simulink model "Mission_Supervisor"  (R2019b)
settings: Solver=FixedStepAuto  StartTime=0.0  StopTime=inf  FixedStep=0.025  RelTol=1e-3  EnableMultiTasking=on
InitFcn:
  | global clientID;
  | clientID=-1;
libraries: dspindex x4
settings Model: EnablePacing=on  Creator=Kleber Cabral  LastModifiedBy=Kleber Cabral
settings DataIOCC: SaveFormat=Array  ReturnWorkspaceOutputs=off
settings OptimizationCC: LifeSpan=inf
settings DebuggingCC: SolverPrmCheckMsg=warning  SFUnexpectedBacktrackingDiag=warning  SFNoUnconditionalDefaultTransitionDiag=warning  ArithmeticOperatorsInVariantConditions=warning
settings HardwareCC: ProdBitPerPointer=32  ProdBitPerSizeT=32  ProdBitPerPtrDiffT=32  ProdLargestAtomicFloat=None  ProdIntDivRoundTo=Undefined  ProdEndianess=Unspecified  ProdWordSize=32  ProdHWDeviceType=32-bit Generic
settings ModelReferenceCC: PropagateSignalLabelsOutOfModel=off
settings SFSimCC: SimUseLocalCustomCode=off  CustomCodeUndefinedFunction=UseInterfaceOnly
settings RTWCC: RTWUseLocalCustomCode=off
settings CodeAppCC: StateflowObjectComments=on
settings GRTTargetCC: TargetLangStandard=C89/C90 (ANSI)  GeneratePreprocessorConditionals=Disable all
settings ConfigComp: CovMetricSettings=dw  CovHtmlReporting=on  CovSaveCumulativeToWorkspaceVar=on  CovSaveSingleToWorkspaceVar=on  CovExternalEMLEnable=off  CovSFcnEnable=off

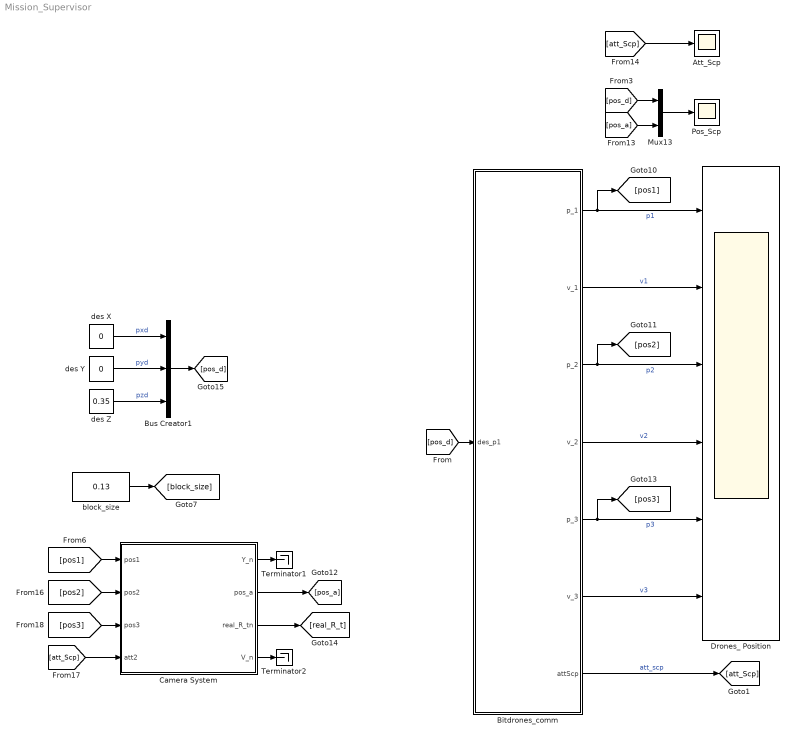
== system Mission_Supervisor ==
  Att_Scp : Scope
  Bitdrones_comm : Subsystem
  Bus Creator1 : BusCreator  Inputs=3
  Camera System : Subsystem
  Drones_ Position : Scope  NumInputPorts=6
  Mux13 : Mux  Inputs=2
  Pos_Scp : Scope
  Terminator1 : Terminator
  Terminator2 : Terminator
  block_size : Constant  Value=0.13
  des X : Constant  Value=0
  des Y : Constant  Value=0
  des Z : Constant  Value=0.35
  wires:
  des X/1 -> Bus Creator1/1  "pxd"
  des Y/1 -> Bus Creator1/2  "pyd"
  des Z/1 -> Bus Creator1/3  "pzd"
  block_size/1 -> [block_size]
  Bitdrones_comm/4(v_2) -> Drones_ Position/4  "v2"
  Bitdrones_comm/2(v_1) -> Drones_ Position/2  "v1"
  Bitdrones_comm/1(p_1) -> [pos1], Drones_ Position/1  "p1"
  Bitdrones_comm/3(p_2) -> [pos2], Drones_ Position/3  "p2"
  Bitdrones_comm/7(attScp) -> [att_Scp]  "att_scp"
  Bitdrones_comm/5(p_3) -> [pos3], Drones_ Position/5  "p3"
  Bitdrones_comm/6(v_3) -> Drones_ Position/6  "v3"
  [att_Scp] -> Att_Scp/1
  [pos_d] -> Mux13/1
  Mux13/1 -> Pos_Scp/1
  [pos_a] -> Mux13/2
  [att_Scp] -> Camera System/4(att2)
  [pos2] -> Camera System/2(pos2)
  Camera System/3(real_R_tn) -> [real_R_t]
  [pos1] -> Camera System/1(pos1)
  [pos3] -> Camera System/3(pos3)
  Camera System/2(pos_a) -> [pos_a]
  Camera System/4(V_n) -> Terminator2/1
  Camera System/1(Y_n) -> Terminator1/1
  Bus Creator1/1 -> [pos_d]
  [pos_d] -> Bitdrones_comm/1(des_p1)

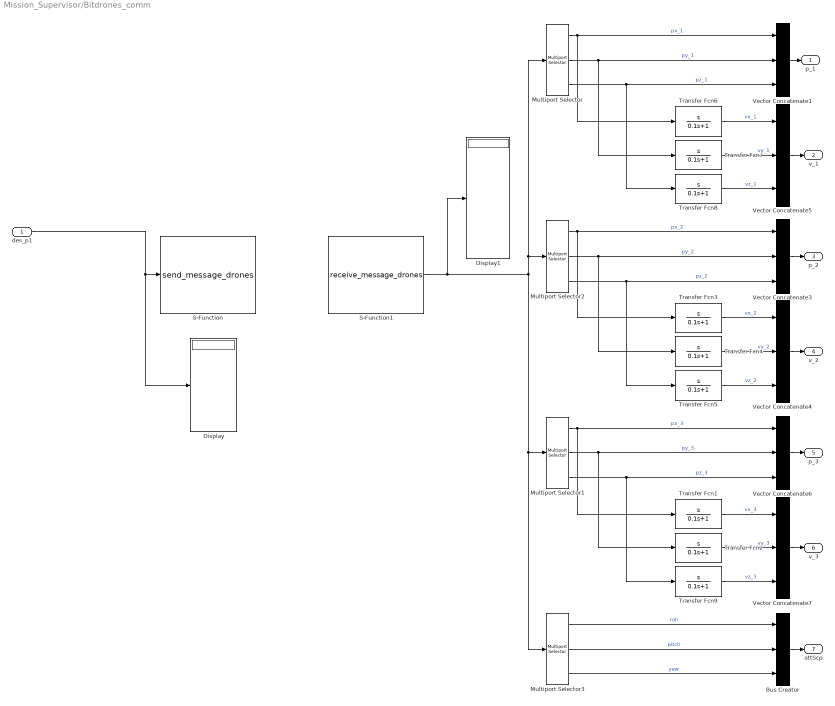
== system Mission_Supervisor/Bitdrones_comm ==
  des_p1 : Inport
  Bus Creator : BusCreator  Inputs=3
  Display : Display
      settings: Decimation=3
  Display1 : Display
      settings: Decimation=3
  Multiport Selector : dspindex/Multiport Selector  rowsOrCols=Rows  idxCellArray={1,2,3}  idxErrMode=Clip Index
  Multiport Selector1 : dspindex/Multiport Selector  rowsOrCols=Rows  idxCellArray={7,8,9}  idxErrMode=Clip Index
  Multiport Selector2 : dspindex/Multiport Selector  rowsOrCols=Rows  idxCellArray={4,5,6}  idxErrMode=Clip Index
  Multiport Selector3 : dspindex/Multiport Selector  rowsOrCols=Rows  idxCellArray={10,11,12}  idxErrMode=Clip Index
  S-Function : S-Function  FunctionName=send_message_drones  SFunctionDeploymentMode=off  EnableBusSupport=off
  S-Function1 : S-Function  FunctionName=receive_message_drones  SFunctionDeploymentMode=off  EnableBusSupport=off
  Transfer Fcn{1..9} (9 alike) : TransferFcn  Numerator=[1 0]  Denominator=[0.1 1]
  Vector Concatenate{1,3..7} (6 alike) : Concatenate  NumInputs=3
  p_1 : Outport
  v_1 : Outport  Port=2
  p_2 : Outport  Port=3
  v_2 : Outport  Port=4
  p_3 : Outport  Port=5
  v_3 : Outport  Port=6
  attScp : Outport  Port=7
  wires:
  Multiport Selector/1 -> Vector Concatenate1/1, Transfer Fcn6/1  "px_1"
  Multiport Selector/2 -> Vector Concatenate1/2, Transfer Fcn7/1  "py_1"
  Multiport Selector/3 -> Vector Concatenate1/3, Transfer Fcn8/1  "pz_1"
  Multiport Selector2/1 -> Vector Concatenate3/1, Transfer Fcn3/1  "px_2"
  Multiport Selector2/2 -> Vector Concatenate3/2, Transfer Fcn4/1  "py_2"
  Multiport Selector2/3 -> Transfer Fcn5/1, Vector Concatenate3/3  "pz_2"
  des_p1/1 -> Display/1, S-Function/1
  Transfer Fcn4/1 -> Vector Concatenate4/2  "vy_2"
  Transfer Fcn5/1 -> Vector Concatenate4/3  "vz_2"
  Vector Concatenate1/1 -> p_1/1
  Vector Concatenate3/1 -> p_2/1
  Vector Concatenate4/1 -> v_2/1
  Transfer Fcn3/1 -> Vector Concatenate4/1  "vx_2"
  Transfer Fcn6/1 -> Vector Concatenate5/1  "vx_1"
  Vector Concatenate5/1 -> v_1/1
  Transfer Fcn8/1 -> Vector Concatenate5/3  "vz_1"
  Transfer Fcn7/1 -> Vector Concatenate5/2  "vy_1"
  Transfer Fcn1/1 -> Vector Concatenate7/1  "vx_3"
  Vector Concatenate7/1 -> v_3/1
  Vector Concatenate6/1 -> p_3/1
  Transfer Fcn9/1 -> Vector Concatenate7/3  "vz_3"
  Transfer Fcn2/1 -> Vector Concatenate7/2  "vy_3"
  Multiport Selector1/3 -> Vector Concatenate6/3, Transfer Fcn9/1  "pz_3"
  Multiport Selector1/2 -> Transfer Fcn2/1, Vector Concatenate6/2  "py_3"
  Multiport Selector1/1 -> Transfer Fcn1/1, Vector Concatenate6/1  "px_3"
  Multiport Selector3/2 -> Bus Creator/2  "pitch"
  Multiport Selector3/3 -> Bus Creator/3  "yaw"
  Bus Creator/1 -> attScp/1
  S-Function1/1 -> Display1/1, Multiport Selector/1, Multiport Selector2/1, Multiport Selector3/1, Multiport Selector1/1
  Multiport Selector3/1 -> Bus Creator/1  "roll"

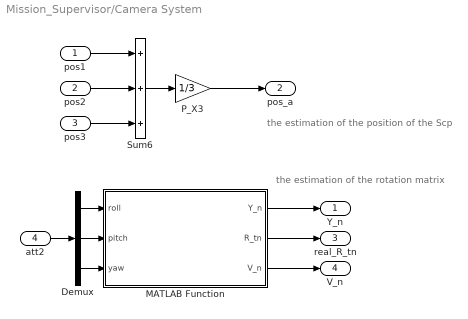
== system Mission_Supervisor/Camera System ==
  note: the estimation of the rotation matrix
  note: the estimation of the position of the Scp
  pos1 : Inport
  pos2 : Inport  Port=2
  pos3 : Inport  Port=3
  att2 : Inport  Port=4
  Demux : Demux  Outputs=3
  MATLAB Function : MATLAB Function  TreatAsAtomicUnit=on
  P_X3 : Gain  Gain=1/3
  Sum6 : Sum  Inputs=+++
  Y_n : Outport  VectorParamsAs1DForOutWhenUnconnected=off
  pos_a : Outport  Port=2  VectorParamsAs1DForOutWhenUnconnected=off
  real_R_tn : Outport  Port=3  VectorParamsAs1DForOutWhenUnconnected=off
  V_n : Outport  Port=4  VectorParamsAs1DForOutWhenUnconnected=off
  wires:
  pos1/1 -> Sum6/1
  pos2/1 -> Sum6/2
  Sum6/1 -> P_X3/1
  P_X3/1 -> pos_a/1
  att2/1 -> Demux/1
  Demux/3 -> MATLAB Function/3(yaw)
  Demux/2 -> MATLAB Function/2(pitch)
  Demux/1 -> MATLAB Function/1(roll)
  MATLAB Function/1(Y_n) -> Y_n/1
  MATLAB Function/2(R_tn) -> real_R_tn/1
  MATLAB Function/3(V_n) -> V_n/1
  pos3/1 -> Sum6/3

== matlab function Mission_Supervisor/Camera System/MATLAB Function ==
  data: roll input; Y_n output; pitch input; yaw input; R_tn output; V_n output
function [Y_n,R_tn,V_n] = EulerAng2RotMat(roll, pitch, yaw)
% a=deg2rad(0);
% b=deg2rad(0);
% c=deg2rad(45);

a=deg2rad(roll);
b=deg2rad(pitch);
c=deg2rad(yaw);

sa=sin(a);ca=cos(a);
sb=sin(b);cb=cos(b);
sc=sin(c);cc=cos(c);
R_tn=[ cc*cb cc*sb*sa-sc*ca cc*sb*ca+sc*sa 
    sc*cb sc*sb*sa+cc*ca sc*sb*ca-cc*sa 
    -sb       cb*sa           cb*ca     ];

%noise of about 1 deg of rotation in each axis
a=deg2rad(0);
b=deg2rad(0);
c=deg2rad(0);
sa=sin(a);ca=cos(a);
sb=sin(b);cb=cos(b);
sc=sin(c);cc=cos(c);
V_n=[ cc*cb cc*sb*sa-sc*ca cc*sb*ca+sc*sa 
    sc*cb sc*sb*sa+cc*ca sc*sb*ca-cc*sa 
    -sb       cb*sa           cb*ca     ];

Y_n = R_tn ;%* V_n;
end
